simulink model "valid"  (Simulink 7.6)
settings: Solver=ode15s  StartTime=0.0  StopTime=10  RelTol=1e-3
undefined symbols (not defined in the file): dd, ddl, nd, ndl
libraries: fl_lib x5, simulink x4, nesl_utility x4, elec_lib x1
CloseFcn:
  | rtwprivate ssgencode ModelCloseRequest System_Model1
settings Model: Creator=Fodi  LastModifiedBy=Fodi

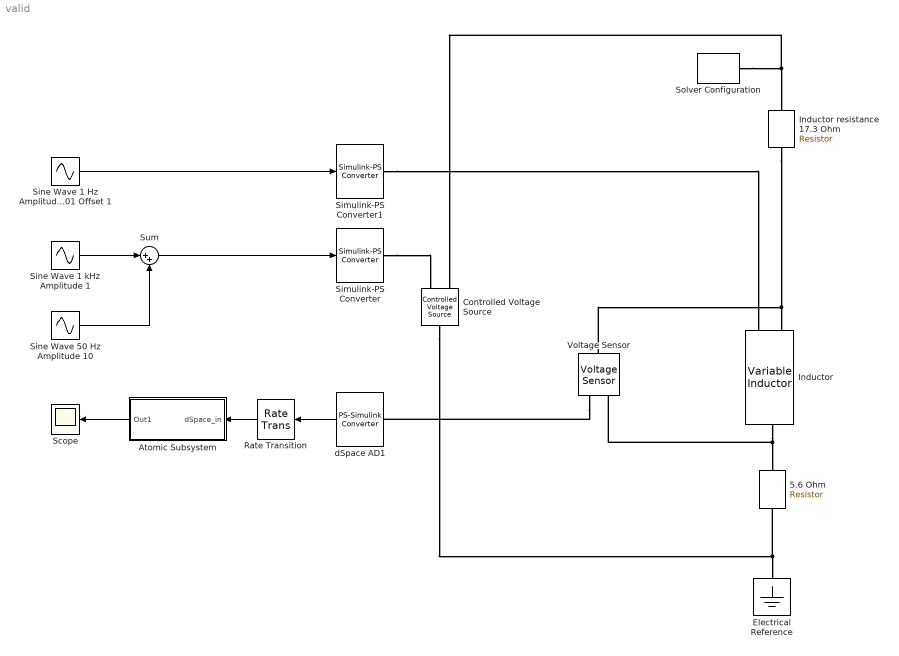
== system valid ==
  5.6 Ohm : fl_lib/Electrical/Electrical Elements/Resistor  DialogController=NetworkEngine.DynNeDlgSource  SystemSampleTime=-1  R=5.6 Ohm  i_Log=off  v_Log=off  LocalVarNames=|i|v  LocalVarDescs=|i|v  LocalVarLogging=[0 0]
  Atomic Subsystem : Subsystem  TreatAsAtomicUnit=on
  Controlled Voltage Source : fl_lib/Electrical/Electrical Sources/Controlled Voltage Source  DialogController=NetworkEngine.DynNeDlgSource  SystemSampleTime=-1  i_Log=off  v_Log=off  LocalVarNames=|i|v  LocalVarDescs=|i|v  LocalVarLogging=[0 0]
  Electrical Reference : fl_lib/Electrical/Electrical Elements/Electrical Reference  DialogController=NetworkEngine.DynNeDlgSource  SystemSampleTime=-1  i_Log=off  LocalVarNames=|i  LocalVarDescs=|i  LocalVarLogging=0
  Inductor : elec_lib/Passive Devices/Variable Inductor  DialogController=NetworkEngine.DynNeDlgSource  SystemSampleTime=-1  prm=2  Lmin=1e-6 H  g=1e-9 1/Ohm  i0=0 A  phi0=0 Wb  LocalVarLogging=[]
  Inductor resistance 17.3 Ohm : fl_lib/Electrical/Electrical Elements/Resistor  DialogController=NetworkEngine.DynNeDlgSource  SystemSampleTime=-1  R=17.3 Ohm  i_Log=off  v_Log=off  LocalVarNames=|i|v  LocalVarDescs=|i|v  LocalVarLogging=[0 0]
  Rate Transition : RateTransition  OutPortSampleTime=0.0001
  Scope : Scope
      settings: YMin=0.002451  YMax=0.0024585
  Simulink-PS Converter : nesl_utility/Simulink-PS Converter  DialogController=NetworkEngine.DynNeUtilDlgSource  SystemSampleTime=-1  PhysicalDomain=network_engine_domain  LeftPortType=input  RightPortType=output  SubClassName=ps_input  Unit=1  AffineConversion=off  InputFilterTimeConstant=.001  UdotUserProvided=0
  Simulink-PS Converter1 : nesl_utility/Simulink-PS Converter  DialogController=NetworkEngine.DynNeUtilDlgSource  SystemSampleTime=-1  PhysicalDomain=network_engine_domain  LeftPortType=input  RightPortType=output  SubClassName=ps_input  Unit=1  AffineConversion=off  InputFilterTimeConstant=.001  UdotUserProvided=0
  Sine Wave 1 Hz Amplitude 0.001 Offset 1 : Sin  SineType=Sample based  Amplitude=0.1  Bias=1  Samples=1000  SampleTime=0.001
  Sine Wave 1 kHz Amplitude 1 : Sin  SineType=Sample based  SampleTime=0.0001
  Sine Wave 50 Hz Amplitude 10 : Sin  SineType=Sample based  Amplitude=10  Bias=2  Frequency=50  Samples=2000  SampleTime=0.0001
  Solver Configuration : nesl_utility/Solver Configuration  DialogController=NetworkEngine.DynNeUtilDlgSource  SystemSampleTime=-1  PhysicalDomain=network_engine_domain  LeftPortType=input  RightPortType=generic  SubClassName=solver  Accelerate=off  Profile=off  ResidualTolerance=1e-9  MaxNonlinIter=3  MaxModeIter=2  DoFixedCost=off  UseLocalSampling=off  DoDC=off  LinearAlgebra=Sparse  LocalSolverSampleTime=.001  LocalSolverChoice=NE_BACKWARD_EULER_ADVANCER  UseLocalSolver=off
  Sum : Sum  Inputs=|++
  Voltage Sensor : fl_lib/Electrical/Electrical Sensors/Voltage Sensor  DialogController=NetworkEngine.DynNeDlgSource  SystemSampleTime=-1  i1_Log=off  v1_Log=off  LocalVarNames=|i1|v1  LocalVarDescs=|i1|v1  LocalVarLogging=[0 0]
  dSpace AD1 : nesl_utility/PS-Simulink Converter  DialogController=NetworkEngine.DynNeUtilDlgSource  SystemSampleTime=-1  PhysicalDomain=network_engine_domain  LeftPortType=input  RightPortType=output  SubClassName=ps_output  Unit=1  AffineConversion=off
  wires:
  Sine Wave 1 kHz Amplitude 1/1 -> Sum/1
  Sine Wave 50 Hz Amplitude 10/1 -> Sum/2
  Sine Wave 1 Hz Amplitude 0.001 Offset 1/1 -> Simulink-PS Converter1/1
  Sum/1 -> Simulink-PS Converter/1
  dSpace AD1/1 -> Rate Transition/1
  Rate Transition/1 -> Atomic Subsystem/1(dSpace_in)
  Atomic Subsystem/1(Out1) -> Scope/1
  connections:
  Controlled Voltage Source/LConn1 -- 5.6 Ohm/RConn1 -- Electrical Reference/LConn1
  Inductor/RConn1 -- 5.6 Ohm/LConn1 -- Voltage Sensor/RConn2
  Simulink-PS Converter/RConn1 -- Controlled Voltage Source/RConn1
  Voltage Sensor/LConn1 -- Inductor/LConn2 -- Inductor resistance 17.3 Ohm/RConn1
  Simulink-PS Converter1/RConn1 -- Inductor/LConn1
  Voltage Sensor/RConn1 -- dSpace AD1/LConn1
  Solver Configuration/RConn1 -- Controlled Voltage Source/RConn2 -- Inductor resistance 17.3 Ohm/LConn1

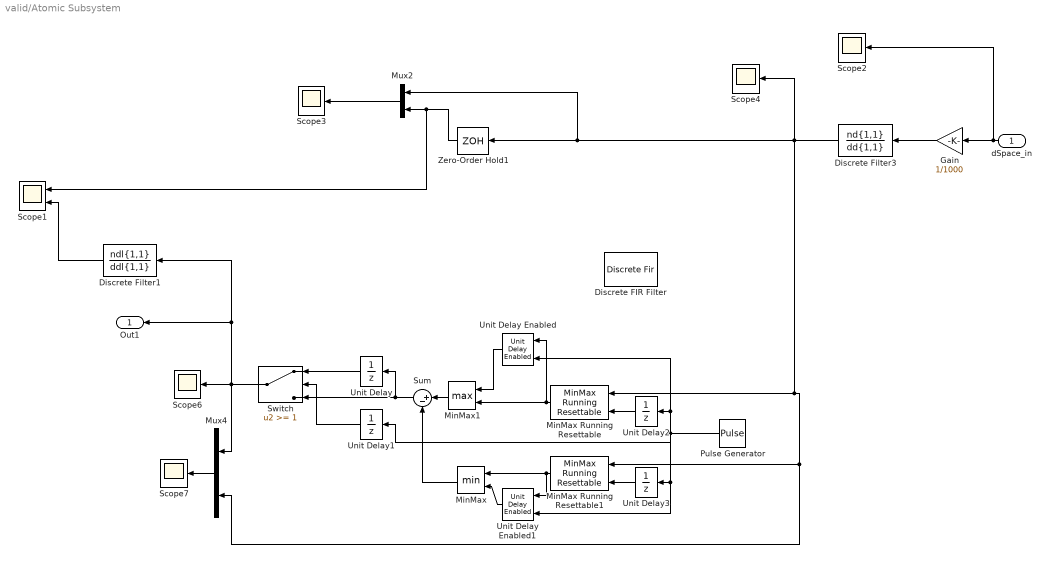
== system valid/Atomic Subsystem ==
  dSpace_in : Inport
  Discrete FIR Filter : DiscreteFir
  Discrete Filter1 : DiscreteFilter  Numerator=ndl{1,1}  Denominator=ddl{1,1}
  Discrete Filter3 : DiscreteFilter  Numerator=nd{1,1}  Denominator=dd{1,1}
  Gain : Gain  Gain=1/1000
  MinMax : MinMax  Inputs=2
  MinMax Running Resettable : simulink/Math Operations/MinMax Running Resettable  SystemSampleTime=-1  Function=max  vinit=0.0
  MinMax Running Resettable1 : simulink/Math Operations/MinMax Running Resettable  SystemSampleTime=-1  Function=min  vinit=0.0
  MinMax1 : MinMax  Function=max  Inputs=2
  Mux2 : Mux  Inputs=2
  Mux4 : Mux  Inputs=2
  Pulse Generator : DiscretePulseGenerator  Period=10  SampleTime=0.001
  Scope1 : Scope  NumInputPorts=2
      settings: TimeRange=3  YMin=0.000495~0.00105825  YMax=0.00056~0.00106075  SaveName=ScopeData2
  Scope{2..4,6..7} (5 alike) : Scope
      Scope2 settings: TimeRange=3  YMin=-0.8  YMax=1  SaveName=ScopeData11
      Scope3 settings: TimeRange=3  YMin=-0.0006  YMax=0.0006  SaveName=ScopeData16
      Scope4 settings: TimeRange=3  YMin=-0.0006  YMax=0.00055  SaveName=ScopeData12
      Scope6 settings: TimeRange=3  YMin=0.001063  YMax=0.001083  SaveName=ScopeData15
      Scope7 settings: TimeRange=3  YMin=-0.0003  YMax=0.0006  SaveName=ScopeData21
  Sum : Sum  Inputs=|+-
  Switch : Switch  Threshold=1
  Unit Delay{,1..3} (4 alike) : UnitDelay  SampleTime=-1
  Unit Delay Enabled : simulink/Additional Math & Discrete/Additional Discrete/Unit Delay Enabled  SystemSampleTime=-1  vinit=0.0  tsamp=-1
  Unit Delay Enabled1 : simulink/Additional Math & Discrete/Additional Discrete/Unit Delay Enabled  SystemSampleTime=-1  vinit=0.0  tsamp=-1
  Zero-Order Hold1 : ZeroOrderHold  SampleTime=1/1000
  Out1 : Outport
  wires:
  dSpace_in/1 -> Scope2/1, Gain/1
  Zero-Order Hold1/1 -> Mux2/2, Scope1/1
  Mux2/1 -> Scope3/1
  Discrete Filter3/1 -> MinMax Running Resettable/1, MinMax Running Resettable1/1, Mux4/2, Scope4/1, Mux2/1, Zero-Order Hold1/1
  MinMax Running Resettable1/1 -> MinMax/1, Unit Delay Enabled1/1
  Pulse Generator/1 -> Unit Delay Enabled/2, Unit Delay2/1, Unit Delay Enabled1/2, Unit Delay3/1, Unit Delay1/1
  Switch/1 -> Scope6/1, Mux4/1, Out1/1, Discrete Filter1/1
  Sum/1 -> Switch/3, Unit Delay/1
  Unit Delay/1 -> Switch/1
  Mux4/1 -> Scope7/1
  MinMax/1 -> Sum/2
  MinMax1/1 -> Sum/1
  MinMax Running Resettable/1 -> MinMax1/2, Unit Delay Enabled/1
  Unit Delay Enabled/1 -> MinMax1/1
  Unit Delay Enabled1/1 -> MinMax/2
  Unit Delay1/1 -> Switch/2
  Unit Delay2/1 -> MinMax Running Resettable/2
  Unit Delay3/1 -> MinMax Running Resettable1/2
  Gain/1 -> Discrete Filter3/1
  Discrete Filter1/1 -> Scope1/2
